simulink model "ERS_sim"  (R2026a)
settings: Solver=ode4  StopTime=30  FixedStep=0.001
InitFcn:
  | % 1. 动态获取当前 .slx 模型文件的存储路径
  | modelPath = get_param(bdroot, 'FileName');
  | 
  | if ~isempty(modelPath)
  |     modelDir = fileparts(modelPath);
  |     % 同时将【当前子系统目录】与【上一层 Power Unit 根目录】加入路径
  |     addpath(modelDir);
  |     addpath(fullfile(modelDir, '..'));
  | end
  | 
  | % 2. 依次加载公共参数与当前子系统参数
  | common_params_init;
  | ers_params_init;
values from neighbouring files (symbols this model uses):
  Battery_Capacity_J = Simulink.Parameter(4000000)    [ers_params_init.m]
  Battery_HeatLossCoeff = Simulink.Parameter(0.05)    [ers_params_init.m]
  Battery_Temp_FaultLim = Simulink.Parameter(55)    [ers_params_init.m]
  Battery_Temp_HighLim = Simulink.Parameter(65)    [ers_params_init.m]
  Battery_Temp_Init_C = Simulink.Parameter(40)    [ers_params_init.m]
  Battery_ThermalMass_JperC = Simulink.Parameter(80000)    [ers_params_init.m]
  Battery_ThermalResistance = Simulink.Parameter(0.02)    [ers_params_init.m]
  ERS_K_Max_Power_W = Simulink.Parameter(350000)    [ers_params_init.m]
  Inertia_Gain = Simulink.Parameter(0.5)    [ers_params_init.m]
  Lap_Deploy_Limit_J_Charge = Simulink.Parameter(4000000)    [ers_params_init.m]
  Lap_Deploy_Limit_J_Push = Simulink.Parameter(12000000)    [ers_params_init.m]
  Lap_Deploy_Limit_J_Race = Simulink.Parameter(8500000)    [ers_params_init.m]
  Lap_Recharge_Limit_J_Charge = Simulink.Parameter(4000000)    [ers_params_init.m]
  Lap_Recharge_Limit_J_Push = Simulink.Parameter(2000000)    [ers_params_init.m]
  Lap_Recharge_Limit_J_Race = Simulink.Parameter(1200000)    [ers_params_init.m]
  MGUK_Power_Boost_W_Charge = Simulink.Parameter(0)    [ers_params_init.m]
  MGUK_Power_Boost_W_Push = Simulink.Parameter(350000)    [ers_params_init.m]
  MGUK_Power_Boost_W_Race = Simulink.Parameter(300000)    [ers_params_init.m]
  MGUK_Power_Regen_W = Simulink.Parameter(250000)    [ers_params_init.m]
  MGUK_Speed_Boost_RPM = Simulink.Parameter(400)    [ers_params_init.m]
  MGUK_Speed_Regen_RPM = Simulink.Parameter(400)    [ers_params_init.m]
  MGUK_Torque_SatLimit = Simulink.Parameter(400)    [ers_params_init.m]
  NonOvertake_Taper_Start_KPH = Simulink.Parameter(290)    [ers_params_init.m]
  Overtake_Energy_Bonus_J = Simulink.Parameter(500000)    [ers_params_init.m]
  Overtake_Full_Power_KPH = Simulink.Parameter(337)    [ers_params_init.m]
  Overtake_Max_Speed_KPH = Simulink.Parameter(355)    [ers_params_init.m]
  Regen_Sign_Gain = Simulink.Parameter(-1)    [ers_params_init.m]
  SOC_Boost_Cutoff = Simulink.Parameter(5)    [ers_params_init.m]
  SOC_Boost_Enter_Charge = Simulink.Parameter(40)    [ers_params_init.m]
  SOC_Boost_Enter_Push = Simulink.Parameter(3)    [ers_params_init.m]
  SOC_Boost_Enter_Race = Simulink.Parameter(7)    [ers_params_init.m]
  SOC_Init_Pct = Simulink.Parameter(50)    [ers_params_init.m]
  SOC_Max_Pct = Simulink.Parameter(100)    [ers_params_init.m]
  SOC_Min_Pct = Simulink.Parameter(0)    [ers_params_init.m]
  SOC_Regen_Cutoff_Charge = Simulink.Parameter(100)    [ers_params_init.m]
  SOC_Regen_Cutoff_Push = Simulink.Parameter(85)    [ers_params_init.m]
  SOC_Regen_Cutoff_Race = Simulink.Parameter(95)    [ers_params_init.m]
  Throttle_Boost_Exit = Simulink.Parameter(75)    [ers_params_init.m]
  Throttle_Boost_Threshold_Charge = Simulink.Parameter(101)    [ers_params_init.m]
  Throttle_Boost_Threshold_Push = Simulink.Parameter(50)    [ers_params_init.m]
  Throttle_Boost_Threshold_Race = Simulink.Parameter(80)    [ers_params_init.m]
  Throttle_Gain = Simulink.Parameter(0.01)    [ers_params_init.m]
  Torque_Cmd_FailSafe_Nm = Simulink.Parameter(0)    [ers_params_init.m]
  Torque_Cmd_Standby_Nm = Simulink.Parameter(0)    [ers_params_init.m]
undefined symbols (not defined in the file or in its folder): Ambient_Temp_C
libraries: simulink_extras x1
settings Model: Creator=nixiaofeng  LastModifiedBy=nixiaofeng
settings SolverCC: ZeroCrossAlgorithm=Adaptive
settings DebuggingCC: IgnoredZcDiagnostic=none  UnderSpecifiedDimensionMsg=warning
settings RTWCC: SystemTargetFile=ert.tlc  CheckMdlBeforeBuild=Warning  Description=Embedded Coder
settings ERTTargetCC: RootIOFormat=Structure reference  GenerateSampleERTMain=on  SupportContinuousTime=on

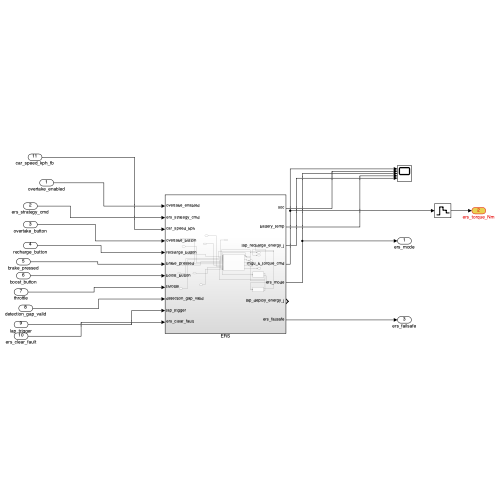
[thumbnail: Simulink's stored preview of the top-level diagram]
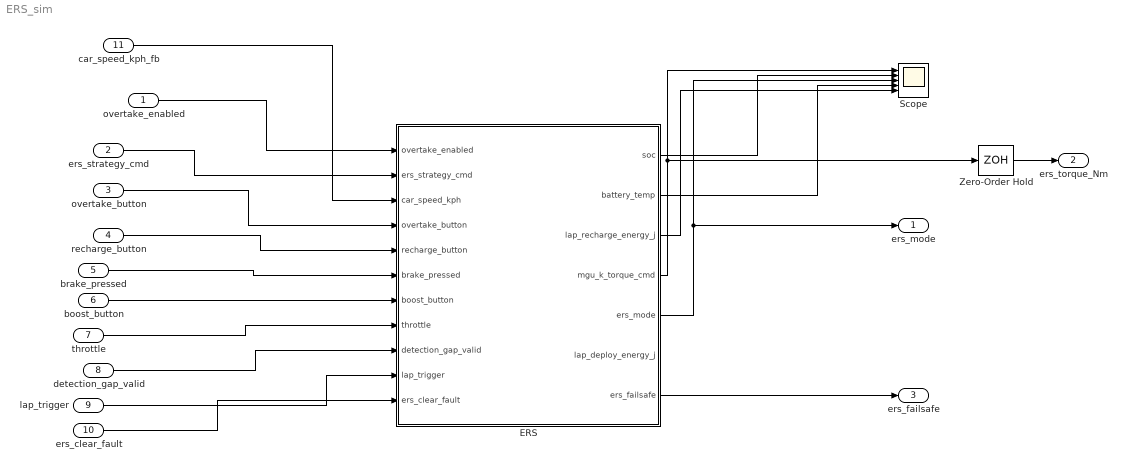
== system ERS_sim ==
  overtake_enabled : Inport  PortDimensions=1
  ers_strategy_cmd : Inport  Port=2  PortDimensions=1
  overtake_button : Inport  Port=3  PortDimensions=1
  recharge_button : Inport  Port=4  PortDimensions=1
  brake_pressed : Inport  Port=5  PortDimensions=1
  boost_button : Inport  Port=6  PortDimensions=1
  throttle : Inport  Port=7  PortDimensions=1
  detection_gap_valid : Inport  Port=8  PortDimensions=1
  lap_trigger : Inport  Port=9  PortDimensions=1
  ers_clear_fault : Inport  Port=10  PortDimensions=1
  car_speed_kph_fb : Inport  Port=11  PortDimensions=1
  ERS : Subsystem
  Scope : Scope  NumInputPorts=5
      settings: ActiveDisplayYMinimum=-81764.7840952557  ActiveDisplayYMaximum=731883.05685730139
  Zero-Order Hold : ZeroOrderHold  SampleTime=-1
  ers_mode : Outport  PortDimensions=1
  ers_torque_Nm : Outport  Port=2  PortDimensions=1
  ers_failsafe : Outport  Port=3  PortDimensions=1
  wires:
  ERS/4(mgu_k_torque_cmd) -> Scope/1, Zero-Order Hold/1
  ERS/5(ers_mode) -> Scope/3, ers_mode/1
  ERS/1(soc) -> Scope/2
  ERS/2(battery_temp) -> Scope/4
  ERS/3(lap_recharge_energy_j) -> Scope/5
  ERS/7(ers_failsafe) -> ers_failsafe/1
  overtake_enabled/1 -> ERS/1(overtake_enabled)
  ers_strategy_cmd/1 -> ERS/2(ers_strategy_cmd)
  overtake_button/1 -> ERS/4(overtake_button)
  recharge_button/1 -> ERS/5(recharge_button)
  brake_pressed/1 -> ERS/6(brake_pressed)
  boost_button/1 -> ERS/7(boost_button)
  throttle/1 -> ERS/8(throttle)
  detection_gap_valid/1 -> ERS/9(detection_gap_valid)
  lap_trigger/1 -> ERS/10(lap_trigger)
  ers_clear_fault/1 -> ERS/11(ers_clear_fault)
  car_speed_kph_fb/1 -> ERS/3(car_speed_kph)
  Zero-Order Hold/1 -> ers_torque_Nm/1

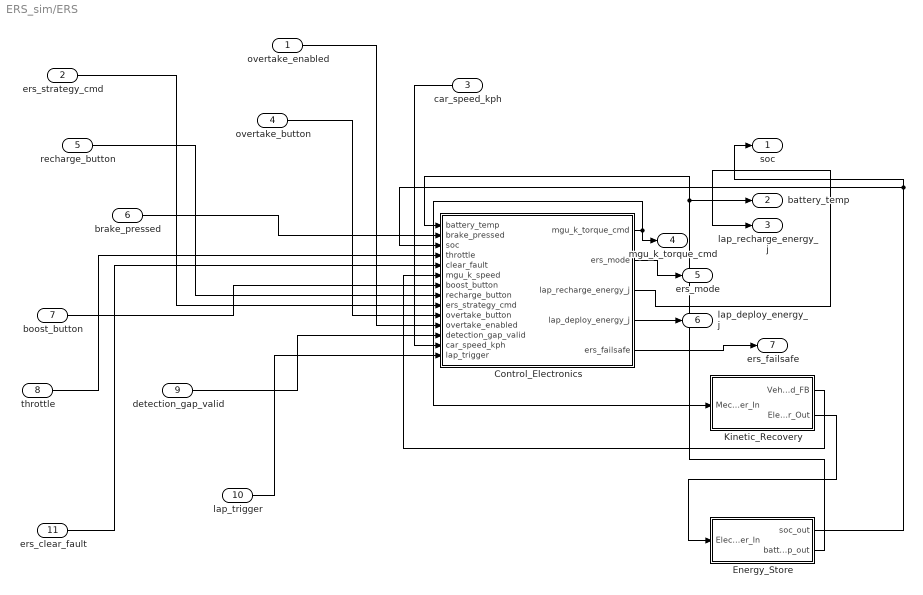
== system ERS_sim/ERS ==
  overtake_enabled : Inport
  ers_strategy_cmd : Inport  Port=2
  car_speed_kph : Inport  Port=3
  overtake_button : Inport  Port=4
  recharge_button : Inport  Port=5
  brake_pressed : Inport  Port=6
  boost_button : Inport  Port=7
  throttle : Inport  Port=8
  detection_gap_valid : Inport  Port=9
  lap_trigger : Inport  Port=10
  ers_clear_fault : Inport  Port=11
  Control_Electronics : Subsystem
  Energy_Store : Subsystem
  Kinetic_Recovery : Subsystem
  soc : Outport
  battery_temp : Outport  Port=2
  lap_recharge_energy_j : Outport  Port=3
  mgu_k_torque_cmd : Outport  Port=4
  ers_mode : Outport  Port=5
  lap_deploy_energy_j : Outport  Port=6
  ers_failsafe : Outport  Port=7
  wires:
  Control_Electronics/4(lap_deploy_energy_j) -> lap_deploy_energy_j/1
  Control_Electronics/1(mgu_k_torque_cmd) -> mgu_k_torque_cmd/1, Kinetic_Recovery/1(Mech_Power_In)
  overtake_enabled/1 -> Control_Electronics/11(overtake_enabled)
  ers_strategy_cmd/1 -> Control_Electronics/9(ers_strategy_cmd)
  detection_gap_valid/1 -> Control_Electronics/12(detection_gap_valid)
  Control_Electronics/3(lap_recharge_energy_j) -> lap_recharge_energy_j/1
  lap_trigger/1 -> Control_Electronics/14(lap_trigger)
  brake_pressed/1 -> Control_Electronics/2(brake_pressed)
  Kinetic_Recovery/2(Elec_Power_Out) -> Energy_Store/1(Elec_Power_In)
  throttle/1 -> Control_Electronics/4(throttle)
  boost_button/1 -> Control_Electronics/7(boost_button)
  Control_Electronics/2(ers_mode) -> ers_mode/1
  overtake_button/1 -> Control_Electronics/10(overtake_button)
  Energy_Store/1(soc_out) -> soc/1, Control_Electronics/3(soc)
  recharge_button/1 -> Control_Electronics/8(recharge_button)
  car_speed_kph/1 -> Control_Electronics/13(car_speed_kph)
  ers_clear_fault/1 -> Control_Electronics/5(clear_fault)
  Kinetic_Recovery/1(Veh_Speed_FB) -> Control_Electronics/6(mgu_k_speed)
  Energy_Store/2(battery_temp_out) -> battery_temp/1, Control_Electronics/1(battery_temp)
  Control_Electronics/5(ers_failsafe) -> ers_failsafe/1

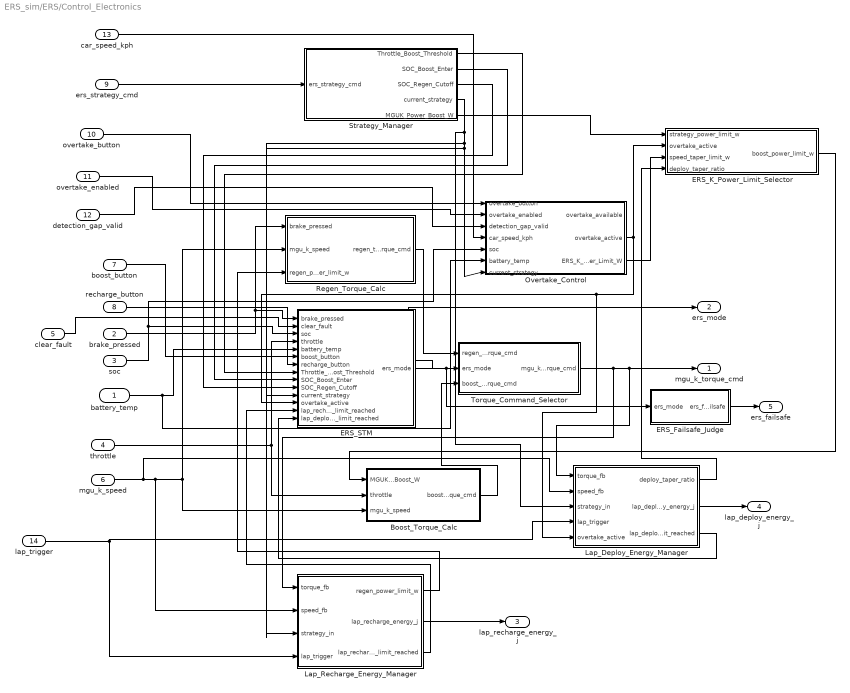
== system ERS_sim/ERS/Control_Electronics ==
  battery_temp : Inport
  brake_pressed : Inport  Port=2
  soc : Inport  Port=3
  throttle : Inport  Port=4
  clear_fault : Inport  Port=5
  mgu_k_speed : Inport  Port=6
  boost_button : Inport  Port=7
  recharge_button : Inport  Port=8
  ers_strategy_cmd : Inport  Port=9
  overtake_button : Inport  Port=10
  overtake_enabled : Inport  Port=11
  detection_gap_valid : Inport  Port=12
  car_speed_kph : Inport  Port=13
  lap_trigger : Inport  Port=14
  Boost_Torque_Calc : Subsystem
  ERS_Failsafe_Judge : Subsystem
  ERS_K_Power_Limit_Selector : Subsystem
  ERS_STM : Stateflow chart  TreatAsAtomicUnit=on
  Lap_Deploy_Energy_Manager : Subsystem
  Lap_Recharge_Energy_Manager : Subsystem
  Overtake_Control : Subsystem
  Regen_Torque_Calc : Subsystem
  Strategy_Manager : Subsystem
  Torque_Command_Selector : Subsystem
  mgu_k_torque_cmd : Outport
  ers_mode : Outport  Port=2
  lap_recharge_energy_j : Outport  Port=3
  lap_deploy_energy_j : Outport  Port=4
  ers_failsafe : Outport  Port=5
  wires:
  ERS_STM/1(ers_mode) -> ERS_Failsafe_Judge/1(ers_mode), Torque_Command_Selector/2(ers_mode), ers_mode/1
  battery_temp/1 -> Overtake_Control/6(battery_temp), ERS_STM/5(battery_temp)
  brake_pressed/1 -> Regen_Torque_Calc/1(brake_pressed), ERS_STM/1(brake_pressed)
  soc/1 -> Overtake_Control/5(soc), ERS_STM/3(soc)
  throttle/1 -> ERS_STM/4(throttle), Boost_Torque_Calc/2(throttle)
  clear_fault/1 -> ERS_STM/2(clear_fault)
  mgu_k_speed/1 -> Lap_Deploy_Energy_Manager/2(speed_fb), Lap_Recharge_Energy_Manager/2(speed_fb), Boost_Torque_Calc/3(mgu_k_speed), Regen_Torque_Calc/2(mgu_k_speed)
  boost_button/1 -> ERS_STM/6(boost_button)
  recharge_button/1 -> ERS_STM/7(recharge_button)
  ers_strategy_cmd/1 -> Strategy_Manager/1(ers_strategy_cmd)
  Strategy_Manager/1(Throttle_Boost_Threshold) -> ERS_STM/8(Throttle_Boost_Threshold)
  Strategy_Manager/2(SOC_Boost_Enter) -> ERS_STM/9(SOC_Boost_Enter)
  Strategy_Manager/3(SOC_Regen_Cutoff) -> ERS_STM/10(SOC_Regen_Cutoff)
  Strategy_Manager/4(current_strategy) -> Lap_Deploy_Energy_Manager/3(strategy_in), Lap_Recharge_Energy_Manager/3(strategy_in), Overtake_Control/7(current_strategy), ERS_STM/11(current_strategy)
  Regen_Torque_Calc/1(regen_torque_cmd) -> Torque_Command_Selector/1(regen_torque_cmd)
  Boost_Torque_Calc/1(boost_torque_cmd) -> Torque_Command_Selector/3(boost_torque_cmd)
  Torque_Command_Selector/1(mgu_k_torque_cmd) -> Lap_Recharge_Energy_Manager/1(torque_fb), Lap_Deploy_Energy_Manager/1(torque_fb), mgu_k_torque_cmd/1
  Overtake_Control/2(overtake_active) -> ERS_K_Power_Limit_Selector/2(overtake_active), Lap_Deploy_Energy_Manager/5(overtake_active), ERS_STM/12(overtake_active)
  overtake_button/1 -> Overtake_Control/1(overtake_button)
  overtake_enabled/1 -> Overtake_Control/2(overtake_enabled)
  detection_gap_valid/1 -> Overtake_Control/3(detection_gap_valid)
  car_speed_kph/1 -> Overtake_Control/4(car_speed_kph)
  Strategy_Manager/5(MGUK_Power_Boost_W) -> ERS_K_Power_Limit_Selector/1(strategy_power_limit_w)
  Overtake_Control/3(ERS_K_Power_Limit_W) -> ERS_K_Power_Limit_Selector/3(speed_taper_limit_w)
  ERS_K_Power_Limit_Selector/1(boost_power_limit_w) -> Boost_Torque_Calc/1(MGUK_Power_Boost_W)
  Lap_Recharge_Energy_Manager/1(regen_power_limit_w) -> Regen_Torque_Calc/3(regen_power_limit_w)
  lap_trigger/1 -> Lap_Recharge_Energy_Manager/4(lap_trigger), Lap_Deploy_Energy_Manager/4(lap_trigger)
  Lap_Recharge_Energy_Manager/2(lap_recharge_energy_j) -> lap_recharge_energy_j/1
  Lap_Recharge_Energy_Manager/3(lap_recharge_limit_reached) -> ERS_STM/13(lap_recharge_limit_reached)
  Lap_Deploy_Energy_Manager/1(deploy_taper_ratio) -> ERS_K_Power_Limit_Selector/4(deploy_taper_ratio)
  Lap_Deploy_Energy_Manager/2(lap_deploy_energy_j) -> lap_deploy_energy_j/1
  Lap_Deploy_Energy_Manager/3(lap_deploy_limit_reached) -> ERS_STM/14(lap_deploy_limit_reached)
  ERS_Failsafe_Judge/1(ers_failsafe) -> ers_failsafe/1

== system ERS_sim/ERS/Energy_Store ==
  Elec_Power_In : Inport
  Battery_SOC : Subsystem
  Battery_Thermal : Subsystem
  soc_out : Outport
  battery_temp_out : Outport  Port=2
  wires:
  Elec_Power_In/1 -> Battery_Thermal/1(Elec_Power_In), Battery_SOC/1(Elec_Power_In)
  Battery_SOC/1(soc_out) -> soc_out/1
  Battery_Thermal/1(battery_temp_out) -> battery_temp_out/1

== system ERS_sim/ERS/Kinetic_Recovery ==
  Mech_Power_In : Inport
  Accel_Calc : Gain  Gain=Inertia_Gain
  Power_calc : Product
  Vehicle_Speed : Integrator  InitialCondition=100
  Veh_Speed_FB : Outport
  Elec_Power_Out : Outport  Port=2
  wires:
  Mech_Power_In/1 -> Accel_Calc/1
  Power_calc/1 -> Elec_Power_Out/1
  Vehicle_Speed/1 -> Power_calc/2, Veh_Speed_FB/1
  Accel_Calc/1 -> Power_calc/1, Vehicle_Speed/1

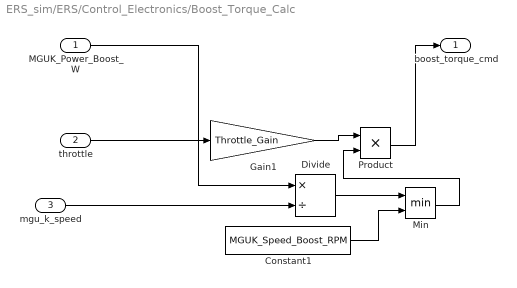
== system ERS_sim/ERS/Control_Electronics/Boost_Torque_Calc ==
  MGUK_Power_Boost_W : Inport
  throttle : Inport  Port=2
  mgu_k_speed : Inport  Port=3
  Constant1 : Constant  Value=MGUK_Speed_Boost_RPM
  Divide : Product  Inputs=*/
  Gain1 : Gain  Gain=Throttle_Gain
  Min : MinMax  Inputs=2
  Product : Product
  boost_torque_cmd : Outport
  wires:
  mgu_k_speed/1 -> Divide/2
  throttle/1 -> Gain1/1
  MGUK_Power_Boost_W/1 -> Divide/1
  Product/1 -> boost_torque_cmd/1
  Constant1/1 -> Min/2
  Divide/1 -> Min/1
  Gain1/1 -> Product/1
  Min/1 -> Product/2

== system ERS_sim/ERS/Control_Electronics/ERS_Failsafe_Judge ==
  ers_mode : Inport
  Constant : Constant
  Equal : RelationalOperator  Operator===  OutDataTypeStr=boolean  RndMeth=Simplest  InputSameDT=off
  ers_failsafe : Outport  OutDataTypeStr=boolean
  wires:
  ers_mode/1 -> Equal/1
  Constant/1 -> Equal/2
  Equal/1 -> ers_failsafe/1

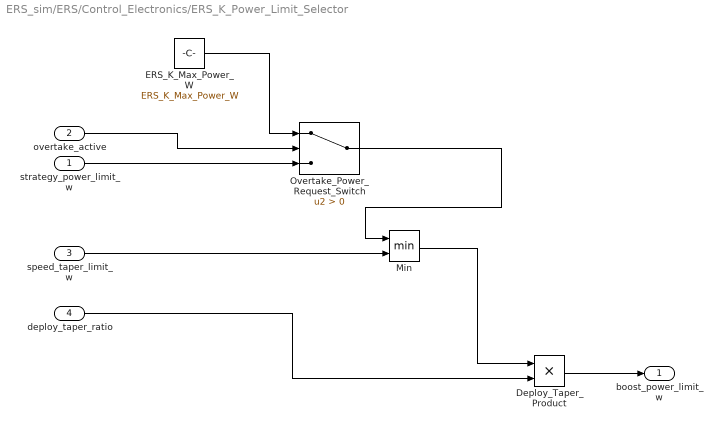
== system ERS_sim/ERS/Control_Electronics/ERS_K_Power_Limit_Selector ==
  strategy_power_limit_w : Inport
  overtake_active : Inport  Port=2
  speed_taper_limit_w : Inport  Port=3
  deploy_taper_ratio : Inport  Port=4
  Deploy_Taper_Product : Product
  ERS_K_Max_Power_W : Constant  Value=ERS_K_Max_Power_W
  Min : MinMax  Inputs=2
  Overtake_Power_Request_Switch : Switch  Criteria=u2 > Threshold  SaturateOnIntegerOverflow=off  InputSameDT=off
  boost_power_limit_w : Outport
  wires:
  ERS_K_Max_Power_W/1 -> Overtake_Power_Request_Switch/1
  overtake_active/1 -> Overtake_Power_Request_Switch/2
  speed_taper_limit_w/1 -> Min/2
  strategy_power_limit_w/1 -> Overtake_Power_Request_Switch/3
  Overtake_Power_Request_Switch/1 -> Min/1
  Min/1 -> Deploy_Taper_Product/1
  deploy_taper_ratio/1 -> Deploy_Taper_Product/2
  Deploy_Taper_Product/1 -> boost_power_limit_w/1

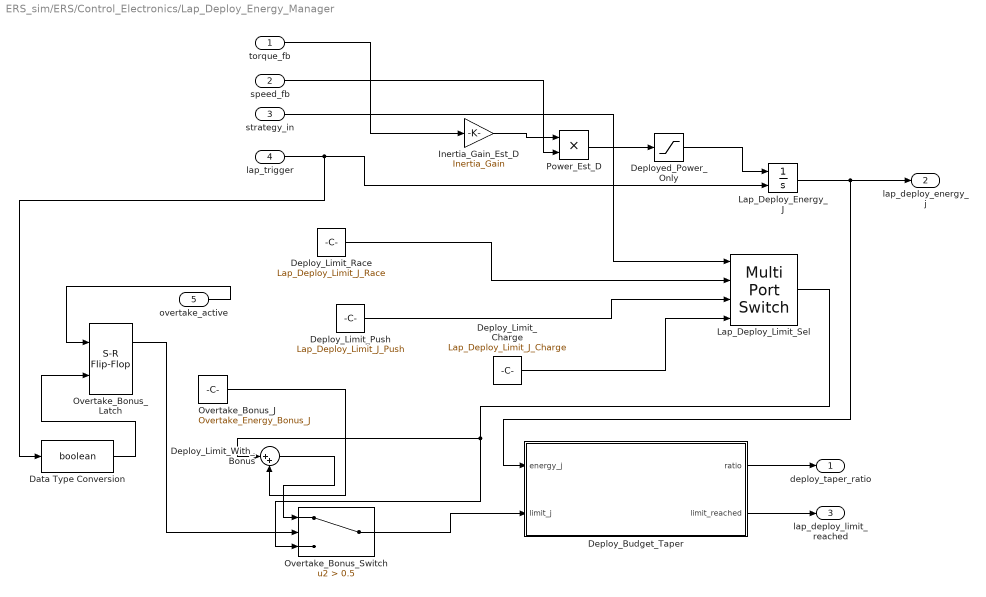
== system ERS_sim/ERS/Control_Electronics/Lap_Deploy_Energy_Manager ==
  torque_fb : Inport
  speed_fb : Inport  Port=2
  strategy_in : Inport  Port=3
  lap_trigger : Inport  Port=4
  overtake_active : Inport  Port=5
  Data Type Conversion : DataTypeConversion  OutDataTypeStr=boolean  SaturateOnIntegerOverflow=off  RndMeth=Floor
  Deploy_Budget_Taper : MATLAB Function  TreatAsAtomicUnit=on
  Deploy_Limit_Charge : Constant  Value=Lap_Deploy_Limit_J_Charge
  Deploy_Limit_Push : Constant  Value=Lap_Deploy_Limit_J_Push
  Deploy_Limit_Race : Constant  Value=Lap_Deploy_Limit_J_Race
  Deploy_Limit_With_Bonus : Sum  Inputs=|++
  Deployed_Power_Only : Saturate  UpperLimit=inf  LowerLimit=0
  Inertia_Gain_Est_D : Gain  Gain=Inertia_Gain
  Lap_Deploy_Energy_J : Integrator  ExternalReset=rising
  Lap_Deploy_Limit_Sel : MultiPortSwitch  DataPortOrder=Zero-based contiguous  zeroidx=on  SaturateOnIntegerOverflow=off  InputSameDT=off
  Overtake_Bonus_J : Constant  Value=Overtake_Energy_Bonus_J
  Overtake_Bonus_Latch : simulink_extras/Flip Flops/S-R Flip-Flop  initial_condition=0
  Overtake_Bonus_Switch : Switch  Criteria=u2 > Threshold  Threshold=0.5  SaturateOnIntegerOverflow=off  InputSameDT=off
  Power_Est_D : Product
  deploy_taper_ratio : Outport
  lap_deploy_energy_j : Outport  Port=2
  lap_deploy_limit_reached : Outport  Port=3
  wires:
  torque_fb/1 -> Inertia_Gain_Est_D/1
  Inertia_Gain_Est_D/1 -> Power_Est_D/1
  speed_fb/1 -> Power_Est_D/2
  Power_Est_D/1 -> Deployed_Power_Only/1
  Deployed_Power_Only/1 -> Lap_Deploy_Energy_J/1
  lap_trigger/1 -> Data Type Conversion/1, Lap_Deploy_Energy_J/2
  strategy_in/1 -> Lap_Deploy_Limit_Sel/1
  Deploy_Limit_Race/1 -> Lap_Deploy_Limit_Sel/2
  Deploy_Limit_Push/1 -> Lap_Deploy_Limit_Sel/3
  Deploy_Limit_Charge/1 -> Lap_Deploy_Limit_Sel/4
  Lap_Deploy_Energy_J/1 -> lap_deploy_energy_j/1, Deploy_Budget_Taper/1(energy_j)
  Lap_Deploy_Limit_Sel/1 -> Overtake_Bonus_Switch/3, Deploy_Limit_With_Bonus/1
  Deploy_Budget_Taper/1(ratio) -> deploy_taper_ratio/1
  Deploy_Budget_Taper/2(limit_reached) -> lap_deploy_limit_reached/1
  Overtake_Bonus_J/1 -> Deploy_Limit_With_Bonus/2
  Deploy_Limit_With_Bonus/1 -> Overtake_Bonus_Switch/1
  Overtake_Bonus_Switch/1 -> Deploy_Budget_Taper/2(limit_j)
  overtake_active/1 -> Overtake_Bonus_Latch/1
  Overtake_Bonus_Latch/1 -> Overtake_Bonus_Switch/2
  Data Type Conversion/1 -> Overtake_Bonus_Latch/2

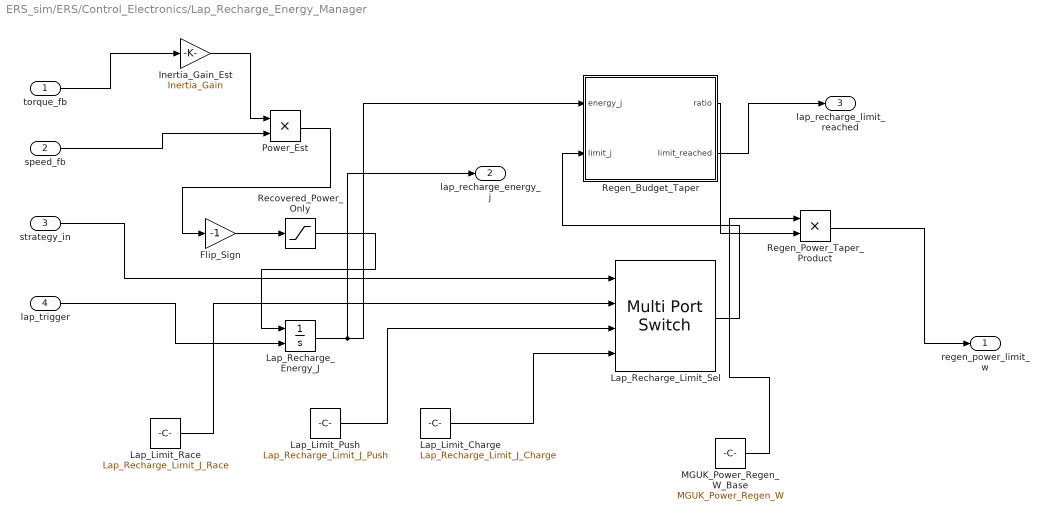
== system ERS_sim/ERS/Control_Electronics/Lap_Recharge_Energy_Manager ==
  torque_fb : Inport
  speed_fb : Inport  Port=2
  strategy_in : Inport  Port=3
  lap_trigger : Inport  Port=4
  Flip_Sign : Gain  Gain=-1
  Inertia_Gain_Est : Gain  Gain=Inertia_Gain
  Lap_Limit_Charge : Constant  Value=Lap_Recharge_Limit_J_Charge
  Lap_Limit_Push : Constant  Value=Lap_Recharge_Limit_J_Push
  Lap_Limit_Race : Constant  Value=Lap_Recharge_Limit_J_Race
  Lap_Recharge_Energy_J : Integrator  ExternalReset=rising  LowerSaturationLimit=0
  Lap_Recharge_Limit_Sel : MultiPortSwitch  DataPortOrder=Zero-based contiguous  zeroidx=on  SaturateOnIntegerOverflow=off  InputSameDT=off
  MGUK_Power_Regen_W_Base : Constant  Value=MGUK_Power_Regen_W
  Power_Est : Product
  Recovered_Power_Only : Saturate  UpperLimit=inf  LowerLimit=0
  Regen_Budget_Taper : MATLAB Function  TreatAsAtomicUnit=on
  Regen_Power_Taper_Product : Product
  regen_power_limit_w : Outport
  lap_recharge_energy_j : Outport  Port=2
  lap_recharge_limit_reached : Outport  Port=3
  wires:
  torque_fb/1 -> Inertia_Gain_Est/1
  Inertia_Gain_Est/1 -> Power_Est/1
  speed_fb/1 -> Power_Est/2
  Power_Est/1 -> Flip_Sign/1
  Flip_Sign/1 -> Recovered_Power_Only/1
  lap_trigger/1 -> Lap_Recharge_Energy_J/2
  Recovered_Power_Only/1 -> Lap_Recharge_Energy_J/1
  strategy_in/1 -> Lap_Recharge_Limit_Sel/1
  Lap_Limit_Race/1 -> Lap_Recharge_Limit_Sel/2
  Lap_Limit_Push/1 -> Lap_Recharge_Limit_Sel/3
  Lap_Limit_Charge/1 -> Lap_Recharge_Limit_Sel/4
  Lap_Recharge_Energy_J/1 -> Regen_Budget_Taper/1(energy_j), lap_recharge_energy_j/1
  Lap_Recharge_Limit_Sel/1 -> Regen_Budget_Taper/2(limit_j)
  Regen_Budget_Taper/2(limit_reached) -> lap_recharge_limit_reached/1
  MGUK_Power_Regen_W_Base/1 -> Regen_Power_Taper_Product/1
  Regen_Budget_Taper/1(ratio) -> Regen_Power_Taper_Product/2
  Regen_Power_Taper_Product/1 -> regen_power_limit_w/1

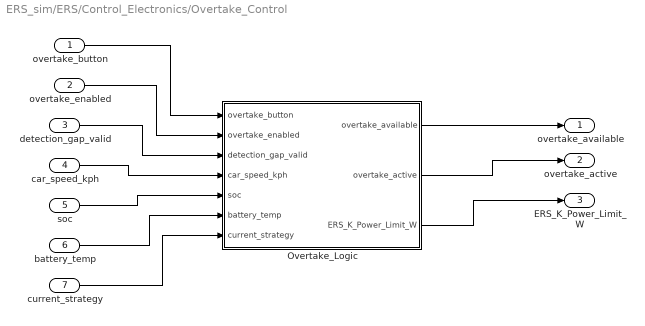
== system ERS_sim/ERS/Control_Electronics/Overtake_Control ==
  overtake_button : Inport
  overtake_enabled : Inport  Port=2
  detection_gap_valid : Inport  Port=3
  car_speed_kph : Inport  Port=4
  soc : Inport  Port=5
  battery_temp : Inport  Port=6
  current_strategy : Inport  Port=7
  Overtake_Logic : MATLAB Function  TreatAsAtomicUnit=on
  overtake_available : Outport
  overtake_active : Outport  Port=2
  ERS_K_Power_Limit_W : Outport  Port=3
  wires:
  overtake_button/1 -> Overtake_Logic/1(overtake_button)
  overtake_enabled/1 -> Overtake_Logic/2(overtake_enabled)
  detection_gap_valid/1 -> Overtake_Logic/3(detection_gap_valid)
  car_speed_kph/1 -> Overtake_Logic/4(car_speed_kph)
  soc/1 -> Overtake_Logic/5(soc)
  battery_temp/1 -> Overtake_Logic/6(battery_temp)
  current_strategy/1 -> Overtake_Logic/7(current_strategy)
  Overtake_Logic/1(overtake_available) -> overtake_available/1
  Overtake_Logic/2(overtake_active) -> overtake_active/1
  Overtake_Logic/3(ERS_K_Power_Limit_W) -> ERS_K_Power_Limit_W/1

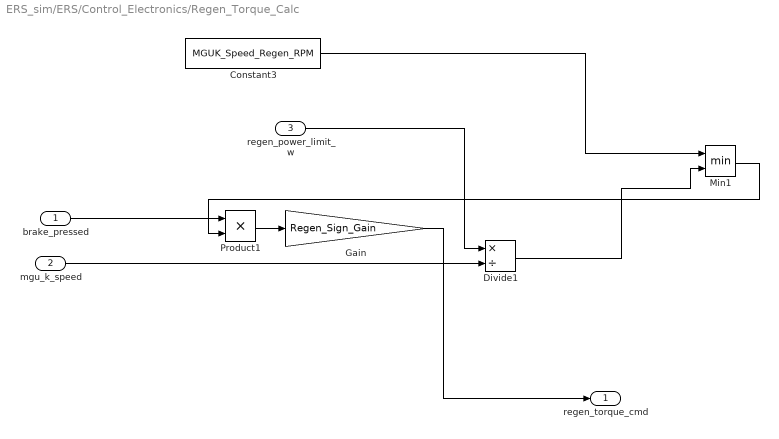
== system ERS_sim/ERS/Control_Electronics/Regen_Torque_Calc ==
  brake_pressed : Inport
  mgu_k_speed : Inport  Port=2
  regen_power_limit_w : Inport  Port=3
  Constant3 : Constant  Value=MGUK_Speed_Regen_RPM
  Divide1 : Product  Inputs=*/
  Gain : Gain  Gain=Regen_Sign_Gain
  Min1 : MinMax  Inputs=2
  Product1 : Product
  regen_torque_cmd : Outport
  wires:
  mgu_k_speed/1 -> Divide1/2
  Divide1/1 -> Min1/2
  Constant3/1 -> Min1/1
  Product1/1 -> Gain/1
  Gain/1 -> regen_torque_cmd/1
  brake_pressed/1 -> Product1/1
  Min1/1 -> Product1/2
  regen_power_limit_w/1 -> Divide1/1

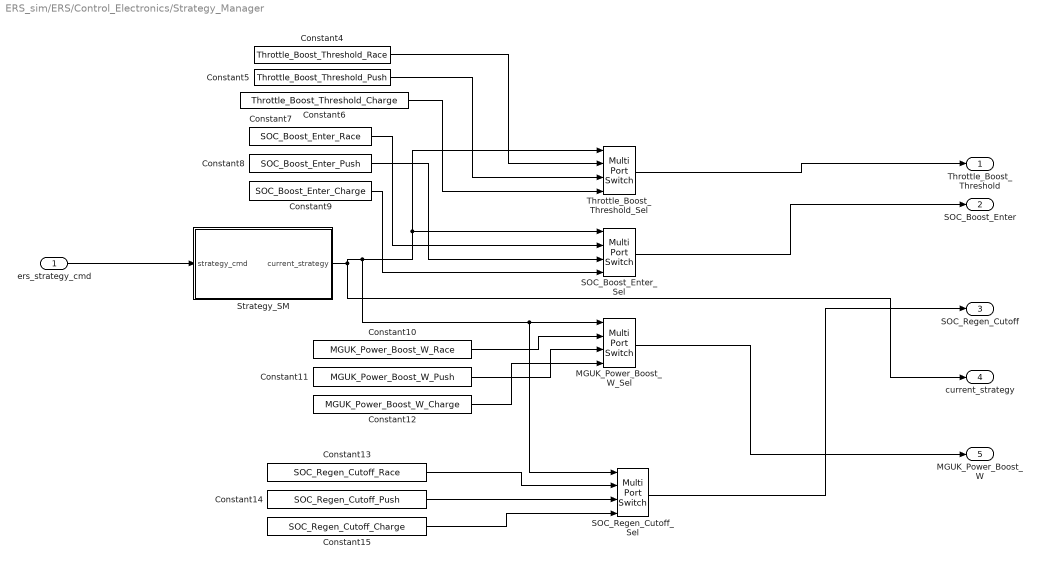
== system ERS_sim/ERS/Control_Electronics/Strategy_Manager ==
  ers_strategy_cmd : Inport
  Constant10 : Constant  Value=MGUK_Power_Boost_W_Race
  Constant11 : Constant  Value=MGUK_Power_Boost_W_Push
  Constant12 : Constant  Value=MGUK_Power_Boost_W_Charge
  Constant13 : Constant  Value=SOC_Regen_Cutoff_Race
  Constant14 : Constant  Value=SOC_Regen_Cutoff_Push
  Constant15 : Constant  Value=SOC_Regen_Cutoff_Charge
  Constant4 : Constant  Value=Throttle_Boost_Threshold_Race
  Constant5 : Constant  Value=Throttle_Boost_Threshold_Push
  Constant6 : Constant  Value=Throttle_Boost_Threshold_Charge
  Constant7 : Constant  Value=SOC_Boost_Enter_Race
  Constant8 : Constant  Value=SOC_Boost_Enter_Push
  Constant9 : Constant  Value=SOC_Boost_Enter_Charge
  MGUK_Power_Boost_W_Sel : MultiPortSwitch  DataPortOrder=Zero-based contiguous  zeroidx=on  SaturateOnIntegerOverflow=off  InputSameDT=off
  SOC_Boost_Enter_Sel : MultiPortSwitch  DataPortOrder=Zero-based contiguous  zeroidx=on  SaturateOnIntegerOverflow=off  InputSameDT=off
  SOC_Regen_Cutoff_Sel : MultiPortSwitch  DataPortOrder=Zero-based contiguous  zeroidx=on  SaturateOnIntegerOverflow=off  InputSameDT=off
  Strategy_SM : Stateflow chart  TreatAsAtomicUnit=on
  Throttle_Boost_Threshold_Sel : MultiPortSwitch  DataPortOrder=Zero-based contiguous  zeroidx=on  SaturateOnIntegerOverflow=off  InputSameDT=off
  Throttle_Boost_Threshold : Outport
  SOC_Boost_Enter : Outport  Port=2
  SOC_Regen_Cutoff : Outport  Port=3
  current_strategy : Outport  Port=4
  MGUK_Power_Boost_W : Outport  Port=5
  wires:
  Constant5/1 -> Throttle_Boost_Threshold_Sel/3
  Constant9/1 -> SOC_Boost_Enter_Sel/4
  Constant4/1 -> Throttle_Boost_Threshold_Sel/2
  SOC_Boost_Enter_Sel/1 -> SOC_Boost_Enter/1
  Constant8/1 -> SOC_Boost_Enter_Sel/3
  MGUK_Power_Boost_W_Sel/1 -> MGUK_Power_Boost_W/1
  Constant14/1 -> SOC_Regen_Cutoff_Sel/3
  Constant13/1 -> SOC_Regen_Cutoff_Sel/2
  SOC_Regen_Cutoff_Sel/1 -> SOC_Regen_Cutoff/1
  Constant12/1 -> MGUK_Power_Boost_W_Sel/4
  Constant11/1 -> MGUK_Power_Boost_W_Sel/3
  Constant10/1 -> MGUK_Power_Boost_W_Sel/2
  Strategy_SM/1(current_strategy) -> SOC_Regen_Cutoff_Sel/1, MGUK_Power_Boost_W_Sel/1, SOC_Boost_Enter_Sel/1, Throttle_Boost_Threshold_Sel/1, current_strategy/1
  Constant6/1 -> Throttle_Boost_Threshold_Sel/4
  ers_strategy_cmd/1 -> Strategy_SM/1(strategy_cmd)
  Constant15/1 -> SOC_Regen_Cutoff_Sel/4
  Constant7/1 -> SOC_Boost_Enter_Sel/2
  Throttle_Boost_Threshold_Sel/1 -> Throttle_Boost_Threshold/1

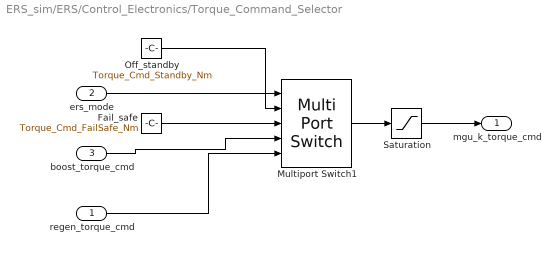
== system ERS_sim/ERS/Control_Electronics/Torque_Command_Selector ==
  regen_torque_cmd : Inport
  ers_mode : Inport  Port=2
  boost_torque_cmd : Inport  Port=3
  Fail_safe : Constant  Value=Torque_Cmd_FailSafe_Nm
  Multiport Switch1 : MultiPortSwitch  DataPortOrder=Zero-based contiguous  Inputs=4  zeroidx=on  SaturateOnIntegerOverflow=off  InputSameDT=off
  Off_standby : Constant  Value=Torque_Cmd_Standby_Nm
  Saturation : Saturate  UpperLimit=MGUK_Torque_SatLimit  LowerLimit=-MGUK_Torque_SatLimit
  mgu_k_torque_cmd : Outport
  wires:
  Off_standby/1 -> Multiport Switch1/2
  Saturation/1 -> mgu_k_torque_cmd/1
  boost_torque_cmd/1 -> Multiport Switch1/4
  Fail_safe/1 -> Multiport Switch1/3
  ers_mode/1 -> Multiport Switch1/1
  regen_torque_cmd/1 -> Multiport Switch1/5
  Multiport Switch1/1 -> Saturation/1

== system ERS_sim/ERS/Energy_Store/Battery_SOC ==
  Elec_Power_In : Inport
  Integrator : Integrator  InitialCondition=SOC_Init_Pct  LimitOutput=on  UpperSaturationLimit=SOC_Max_Pct  LowerSaturationLimit=SOC_Min_Pct
  Power_to_SOC_rate : Gain  Gain=-100/Battery_Capacity_J
  soc_out : Outport
  wires:
  Integrator/1 -> soc_out/1
  Elec_Power_In/1 -> Power_to_SOC_rate/1
  Power_to_SOC_rate/1 -> Integrator/1

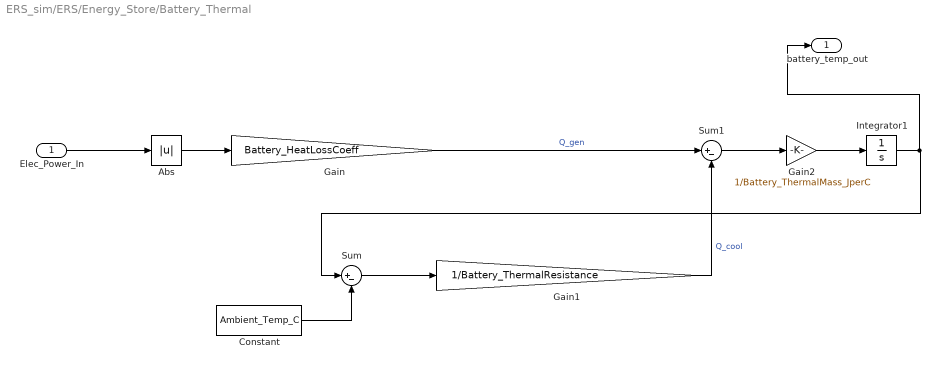
== system ERS_sim/ERS/Energy_Store/Battery_Thermal ==
  Elec_Power_In : Inport
  Abs : Abs  SaturateOnIntegerOverflow=off
  Constant : Constant  Value=Ambient_Temp_C
  Gain : Gain  Gain=Battery_HeatLossCoeff
  Gain1 : Gain  Gain=1/Battery_ThermalResistance
  Gain2 : Gain  Gain=1/Battery_ThermalMass_JperC
  Integrator1 : Integrator  InitialCondition=Battery_Temp_Init_C
  Sum : Sum  Inputs=|+-
  Sum1 : Sum  Inputs=|+-
  battery_temp_out : Outport
  wires:
  Gain2/1 -> Integrator1/1
  Integrator1/1 -> battery_temp_out/1, Sum/1
  Gain/1 -> Sum1/1  "Q_gen"
  Abs/1 -> Gain/1
  Gain1/1 -> Sum1/2  "Q_cool"
  Constant/1 -> Sum/2
  Sum1/1 -> Gain2/1
  Elec_Power_In/1 -> Abs/1
  Sum/1 -> Gain1/1

== matlab function ERS_sim/ERS/Control_Electronics/Lap_Recharge_Energy_Manager/Regen_Budget_Taper ==
  data: energy_j input; ratio output; limit_j input; limit_reached output
function [ratio, limit_reached] = fcn(energy_j, limit_j)
%#codegen
margin_frac = 0.1;              % 剩余预算低于10%时开始线性衰减，可调
taper_band  = margin_frac * limit_j;
remaining   = limit_j - energy_j;

if taper_band <= 0
    % limit_j 异常为0或负数时的保护，避免除零
    if remaining <= 0
        ratio = 0; limit_reached = 1;
    else
        ratio = 1; limit_reached = 0;
    end
elseif remaining <= 0
    ratio = 0; limit_reached = 1;
elseif remaining >= taper_band
    ratio = 1; limit_reached = 0;
else
    ratio = remaining / taper_band;
    limit_reached = 0;
end

== matlab function ERS_sim/ERS/Control_Electronics/Lap_Deploy_Energy_Manager/Deploy_Budget_Taper ==
  data: energy_j input; ratio output; limit_j input; limit_reached output
function [ratio, limit_reached] = fcn(energy_j, limit_j)
%#codegen
margin_frac = 0.1;              % 剩余预算低于10%时开始线性衰减，可调
taper_band  = margin_frac * limit_j;
remaining   = limit_j - energy_j;

if taper_band <= 0
    % limit_j 异常为0或负数时的保护，避免除零
    if remaining <= 0
        ratio = 0; limit_reached = 1;
    else
        ratio = 1; limit_reached = 0;
    end
elseif remaining <= 0
    ratio = 0; limit_reached = 1;
elseif remaining >= taper_band
    ratio = 1; limit_reached = 0;
else
    ratio = remaining / taper_band;
    limit_reached = 0;
end

== stateflow chart ERS_sim/ERS/Control_Electronics/Strategy_Manager/Strategy_SM ==
  state Race
    entry: current_strategy = 0;
  state Push
    entry: current_strategy = 1;
  state Charge
    entry: current_strategy = 2;
  (default) -> Race
  Charge -> Race [order 2] : [strategy_cmd == 0]
  Race -> Push [order 1] : [strategy_cmd == 1]
  Push -> Race [order 1] : [strategy_cmd == 0]
  Race -> Charge [order 2] : [strategy_cmd == 2]
  Charge -> Push [order 1] : [strategy_cmd == 1]
  Push -> Charge [order 2] : [strategy_cmd == 2]
  data: strategy_cmd input; current_strategy output

== matlab function ERS_sim/ERS/Control_Electronics/Overtake_Control/Overtake_Logic ==
  data: overtake_button input; overtake_available output; overtake_enabled input; detection_gap_valid input; car_speed_kph input; soc input; battery_temp input; current_strategy input; overtake_active output; ERS_K_Power_Limit_W output; SOC_Boost_Cutoff parameter; Battery_Temp_HighLim parameter; Overtake_Full_Power_KPH parameter; Overtake_Max_Speed_KPH parameter; NonOvertake_Taper_Start_KPH parameter; ERS_K_Max_Power_W parameter
function [overtake_available, overtake_active, ERS_K_Power_Limit_W] = ...
    OvertakeLogic(overtake_button, overtake_enabled, detection_gap_valid, ...
                  car_speed_kph, soc, battery_temp, current_strategy, SOC_Boost_Cutoff, Battery_Temp_HighLim, Overtake_Full_Power_KPH, Overtake_Max_Speed_KPH, NonOvertake_Taper_Start_KPH, ERS_K_Max_Power_W)

% Charge strategy = 2 时禁止超车部署；如果你想允许 Charge 下强制超车，删掉这一项。
strategy_allows = current_strategy ~= 2;

system_ok = soc > SOC_Boost_Cutoff && battery_temp < Battery_Temp_HighLim;

overtake_available = overtake_enabled && detection_gap_valid && ...
                     strategy_allows && system_ok;

overtake_active = overtake_available && overtake_button;

v = car_speed_kph;

if overtake_active
    if v <= Overtake_Full_Power_KPH
        p_kw = 350;
    elseif v < Overtake_Max_Speed_KPH
        p_kw = 350 * (Overtake_Max_Speed_KPH - v) / ...
               (Overtake_Max_Speed_KPH - Overtake_Full_Power_KPH);
    else
        p_kw = 0;
    end
else
    if v <= NonOvertake_Taper_Start_KPH
        p_kw = 350;
    elseif v < Overtake_Max_Speed_KPH
        p_kw = 350 * (Overtake_Max_Speed_KPH - v) / ...
               (Overtake_Max_Speed_KPH - NonOvertake_Taper_Start_KPH);
    else
        p_kw = 0;
    end
end

ERS_K_Power_Limit_W = max(0, min(p_kw * 1000, ERS_K_Max_Power_W));
end

== stateflow chart ERS_sim/ERS/Control_Electronics/ERS_STM ==
  state Off_Standby_State
    entry: ers_mode = 0;
  state Boost_State
    entry: ers_mode = 2;
  state Regen_State
    entry: ers_mode = 3;
  state Fail_Safe_State
    entry: ers_mode = 1;
  (default) -> Off_Standby_State
  Boost_State -> Off_Standby_State [order 1] : [(boost_button == 0&&overtake_active == 0) || throttle<=Throttle_Boost_Exit || soc<=SOC_Boost_Cutoff || current_strategy ==2 || lap_deploy_limit_reached==1]
  Regen_State -> Off_Standby_State [order 1] : [recharge_button == 0 || brake_pressed == 0 || (soc >= SOC_Max_Pct && battery_temp <= Battery_Temp_HighLim) || lap_recharge_limit_reached==1]
  Off_Standby_State -> Boost_State [order 1] : [(boost_button == 1 || overtake_active == 1) && current_strategy ~= 2 && throttle > Throttle_Boost_Threshold && soc > SOC_Boost_Enter  && lap_deploy_limit_reached==0]
  Fail_Safe_State -> Off_Standby_State : [clear_fault==1 && battery_temp<Battery_Temp_FaultLim]
  Off_Standby_State -> Regen_State [order 2] : [recharge_button == 1 && brake_pressed == 1 && soc < SOC_Regen_Cutoff && lap_recharge_limit_reached==0]
  Boost_State -> Fail_Safe_State [order 2] : [battery_temp>Battery_Temp_HighLim || soc>=SOC_Max_Pct]
  Regen_State -> Fail_Safe_State [order 2] : [battery_temp>Battery_Temp_HighLim || soc>=SOC_Max_Pct]
  data: brake_pressed input; clear_fault input; soc input; throttle input; ers_mode output; battery_temp input; SOC_Boost_Cutoff parameter; SOC_Max_Pct parameter; Battery_Temp_HighLim parameter; Battery_Temp_FaultLim parameter; boost_button input; recharge_button input; Throttle_Boost_Exit parameter; Throttle_Boost_Threshold input; SOC_Boost_Enter input; SOC_Regen_Cutoff input; current_strategy input; overtake_active input; lap_recharge_limit_reached input; lap_deploy_limit_reached input
